simulink model "plant_fullstate"  (R2021b)
settings: Solver=VariableStepAuto  StartTime=0.0  StopTime=10.0  RelTol=1e-3
values from neighbouring files (symbols this model uses):
  Kx = [27.3799665179 22.9258092854 0.383652278901]    [gain_matrix.mat]    (also in pole_placement.m = [Kgain_x(1 : 2), Kgain_x(4)])
undefined symbols (not defined in the file or in its folder): A, B, C, D, Ki
settings Model: Creator=eduar  LastModifiedBy=eduar

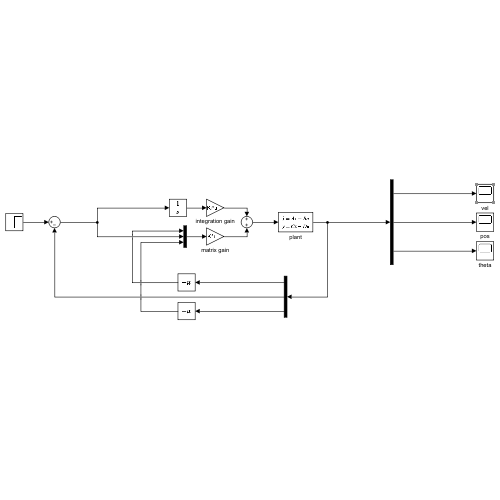
[thumbnail: Simulink's stored preview of the top-level diagram]
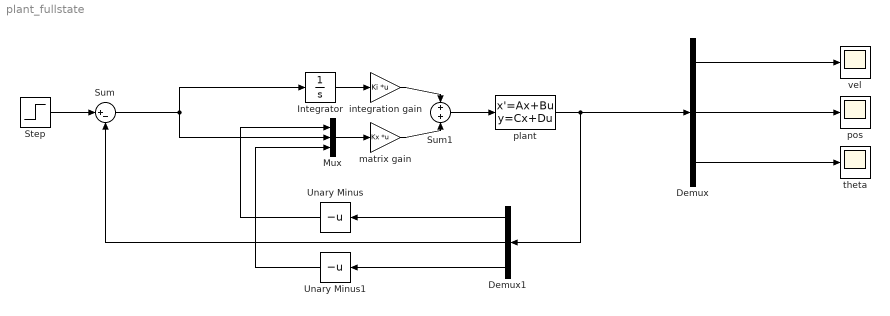
== system plant_fullstate ==
  Demux : Demux  Outputs=3
  Demux1 : Demux  Outputs=3
  Integrator : Integrator
  Mux : Mux  Inputs=3
  Step : Step  Time=0  SampleTime=0
  Sum : Sum  Inputs=|+-
  Sum1 : Sum  Inputs=+|+
  Unary Minus : UnaryMinus
  Unary Minus1 : UnaryMinus
  integration gain : Gain  Gain=Ki  Multiplication=Matrix(K*u)
  matrix gain : Gain  Gain=Kx  Multiplication=Matrix(K*u)
  plant : StateSpace  A=A  B=B  C=C  D=D  InitialCondition=0
  pos : Scope
  theta : Scope
  vel : Scope
  wires:
  plant/1 -> Demux1/1, Demux/1
  Demux/2 -> pos/1
  Demux/1 -> vel/1
  Demux/3 -> theta/1
  Demux1/2 -> Sum/2
  Step/1 -> Sum/1
  Sum/1 -> Mux/2, Integrator/1
  Mux/1 -> matrix gain/1
  Integrator/1 -> integration gain/1
  integration gain/1 -> Sum1/1
  matrix gain/1 -> Sum1/2
  Sum1/1 -> plant/1
  Demux1/1 -> Unary Minus/1
  Demux1/3 -> Unary Minus1/1
  Unary Minus/1 -> Mux/1
  Unary Minus1/1 -> Mux/3
